simulink model "CATSS_Physical_ServiceCorePods"  (R2026a)
settings: Solver=VariableStepAuto
settings Model: DataDictionary=CATSS_PhysicalInterfaces.sldd  Creator=sdagen  LastModifiedBy=sdagen

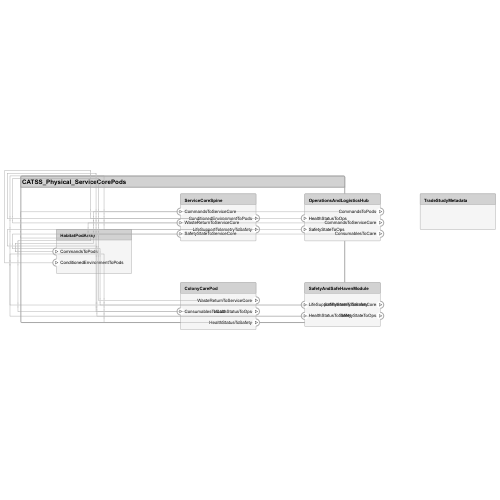
[thumbnail: Simulink's stored preview of the top-level diagram]
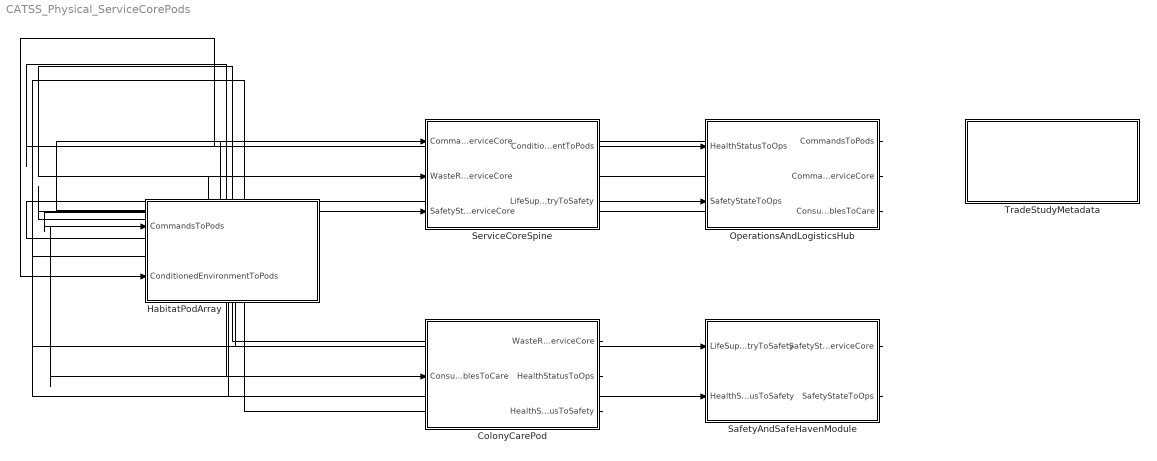
== system CATSS_Physical_ServiceCorePods ==
  ColonyCarePod : Subsystem
      settings: PortSchema="{\"entries\":[{\"content\":{\"headerSize\":26,\"margin\":15,\"minimumSpacing\":25,\"sides\":[{\"content\":{\"connectorIds\":[\"In1\"]},\"type\":\"ConnectorPlacement.EquallySpacedRectSide\",\"uuid\":\"fac29802-5ea5-4ebb-a4ed-86ec77815f5f\"},{\"content\":{\"connectorIds\":[\"Out1\",\"Out2\",\"Out3\"],\"side\":\"RIGHT\"},\"type\":\"ConnectorPlacement.EquallySpacedRectSide\",\"uuid\":\"7714f217-6bf1-4c7c-9160-bb80ade3ec0d\"},{\"content\":{\"side\":\"TOP\"},\"type\":\"ConnectorPlacement.EquallySpacedRectSide\",\"uuid\":\"21f04823-5172-4490-ad65-82ec45233f3c\"}]},\"type\":\"ConnectorPlacement.EquallySpacedConnector\",\"uuid\":\"7a688d36-5efc-41ce-92bb-92fe971cf983\"}],\"packageUris\":[\"http://schema.mathworks.com/mf0/Connector/R2020b\"],\"version\":\"1.0\"}"
  HabitatPodArray : Subsystem
      settings: PortSchema="{\"entries\":[{\"content\":{\"headerSize\":26,\"margin\":15,\"minimumSpacing\":25,\"sides\":[{\"content\":{\"connectorIds\":[\"In1\",\"In2\"]},\"type\":\"ConnectorPlacement.EquallySpacedRectSide\",\"uuid\":\"fac29802-5ea5-4ebb-a4ed-86ec77815f5f\"},{\"content\":{\"side\":\"RIGHT\"},\"type\":\"ConnectorPlacement.EquallySpacedRectSide\",\"uuid\":\"7714f217-6bf1-4c7c-9160-bb80ade3ec0d\"},{\"content\":{\"side\":\"TOP\"},\"type\":\"ConnectorPlacement.EquallySpacedRectSide\",\"uuid\":\"21f04823-5172-4490-ad65-82ec45233f3c\"}]},\"type\":\"ConnectorPlacement.EquallySpacedConnector\",\"uuid\":\"7a688d36-5efc-41ce-92bb-92fe971cf983\"}],\"packageUris\":[\"http://schema.mathworks.com/mf0/Connector/R2020b\"],\"version\":\"1.0\"}"
  OperationsAndLogisticsHub : Subsystem
      settings: PortSchema="{\"entries\":[{\"content\":{\"headerSize\":26,\"margin\":15,\"minimumSpacing\":25,\"sides\":[{\"content\":{\"connectorIds\":[\"In1\",\"In2\"]},\"type\":\"ConnectorPlacement.EquallySpacedRectSide\",\"uuid\":\"fac29802-5ea5-4ebb-a4ed-86ec77815f5f\"},{\"content\":{\"connectorIds\":[\"Out1\",\"Out2\",\"Out3\"],\"side\":\"RIGHT\"},\"type\":\"ConnectorPlacement.EquallySpacedRectSide\",\"uuid\":\"7714f217-6bf1-4c7c-9160-bb80ade3ec0d\"},{\"content\":{\"side\":\"TOP\"},\"type\":\"ConnectorPlacement.EquallySpacedRectSide\",\"uuid\":\"21f04823-5172-4490-ad65-82ec45233f3c\"}]},\"type\":\"ConnectorPlacement.EquallySpacedConnector\",\"uuid\":\"7a688d36-5efc-41ce-92bb-92fe971cf983\"}],\"packageUris\":[\"http://schema.mathworks.com/mf0/Connector/R2020b\"],\"version\":\"1.0\"}"
  SafetyAndSafeHavenModule : Subsystem
      settings: PortSchema="{\"entries\":[{\"content\":{\"headerSize\":26,\"margin\":15,\"minimumSpacing\":25,\"sides\":[{\"content\":{\"connectorIds\":[\"In1\",\"In2\"]},\"type\":\"ConnectorPlacement.EquallySpacedRectSide\",\"uuid\":\"fac29802-5ea5-4ebb-a4ed-86ec77815f5f\"},{\"content\":{\"connectorIds\":[\"Out1\",\"Out2\"],\"side\":\"RIGHT\"},\"type\":\"ConnectorPlacement.EquallySpacedRectSide\",\"uuid\":\"7714f217-6bf1-4c7c-9160-bb80ade3ec0d\"},{\"content\":{\"side\":\"TOP\"},\"type\":\"ConnectorPlacement.EquallySpacedRectSide\",\"uuid\":\"21f04823-5172-4490-ad65-82ec45233f3c\"}]},\"type\":\"ConnectorPlacement.EquallySpacedConnector\",\"uuid\":\"7a688d36-5efc-41ce-92bb-92fe971cf983\"}],\"packageUris\":[\"http://schema.mathworks.com/mf0/Connector/R2020b\"],\"version\":\"1.0\"}"
  ServiceCoreSpine : Subsystem
      settings: PortSchema="{\"entries\":[{\"content\":{\"headerSize\":26,\"margin\":15,\"minimumSpacing\":25,\"sides\":[{\"content\":{\"connectorIds\":[\"In1\",\"In2\",\"In3\"]},\"type\":\"ConnectorPlacement.EquallySpacedRectSide\",\"uuid\":\"fac29802-5ea5-4ebb-a4ed-86ec77815f5f\"},{\"content\":{\"connectorIds\":[\"Out1\",\"Out2\"],\"side\":\"RIGHT\"},\"type\":\"ConnectorPlacement.EquallySpacedRectSide\",\"uuid\":\"7714f217-6bf1-4c7c-9160-bb80ade3ec0d\"},{\"content\":{\"side\":\"TOP\"},\"type\":\"ConnectorPlacement.EquallySpacedRectSide\",\"uuid\":\"21f04823-5172-4490-ad65-82ec45233f3c\"}]},\"type\":\"ConnectorPlacement.EquallySpacedConnector\",\"uuid\":\"7a688d36-5efc-41ce-92bb-92fe971cf983\"}],\"packageUris\":[\"http://schema.mathworks.com/mf0/Connector/R2020b\"],\"version\":\"1.0\"}"
  TradeStudyMetadata : Subsystem
      settings: PortSchema="{\"entries\":[{\"content\":{\"headerSize\":26,\"margin\":15,\"minimumSpacing\":25,\"sides\":[{\"content\":{},\"type\":\"ConnectorPlacement.EquallySpacedRectSide\",\"uuid\":\"fac29802-5ea5-4ebb-a4ed-86ec77815f5f\"},{\"content\":{\"side\":\"RIGHT\"},\"type\":\"ConnectorPlacement.EquallySpacedRectSide\",\"uuid\":\"7714f217-6bf1-4c7c-9160-bb80ade3ec0d\"},{\"content\":{\"side\":\"TOP\"},\"type\":\"ConnectorPlacement.EquallySpacedRectSide\",\"uuid\":\"21f04823-5172-4490-ad65-82ec45233f3c\"}]},\"type\":\"ConnectorPlacement.EquallySpacedConnector\",\"uuid\":\"7a688d36-5efc-41ce-92bb-92fe971cf983\"}],\"packageUris\":[\"http://schema.mathworks.com/mf0/Connector/R2020b\"],\"version\":\"1.0\"}"
  wires:
  OperationsAndLogisticsHub/1(CommandsToPods) -> HabitatPodArray/1(CommandsToPods)
  OperationsAndLogisticsHub/2(CommandsToServiceCore) -> ServiceCoreSpine/1(CommandsToServiceCore)
  OperationsAndLogisticsHub/3(ConsumablesToCare) -> ColonyCarePod/1(ConsumablesToCare)
  ServiceCoreSpine/1(ConditionedEnvironmentToPods) -> HabitatPodArray/2(ConditionedEnvironmentToPods)
  ServiceCoreSpine/2(LifeSupportTelemetryToSafety) -> SafetyAndSafeHavenModule/1(LifeSupportTelemetryToSafety)
  ColonyCarePod/1(WasteReturnToServiceCore) -> ServiceCoreSpine/2(WasteReturnToServiceCore)
  ColonyCarePod/2(HealthStatusToOps) -> OperationsAndLogisticsHub/1(HealthStatusToOps)
  ColonyCarePod/3(HealthStatusToSafety) -> SafetyAndSafeHavenModule/2(HealthStatusToSafety)
  SafetyAndSafeHavenModule/1(SafetyStateToServiceCore) -> ServiceCoreSpine/3(SafetyStateToServiceCore)
  SafetyAndSafeHavenModule/2(SafetyStateToOps) -> OperationsAndLogisticsHub/2(SafetyStateToOps)

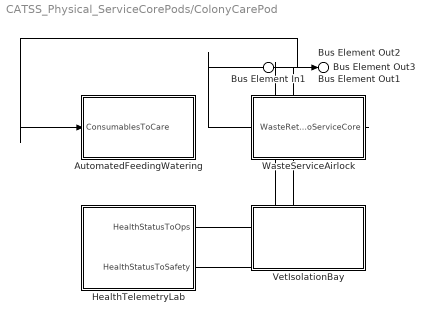
== system CATSS_Physical_ServiceCorePods/ColonyCarePod ==
  Bus Element In1 : Inport  PortName=ConsumablesToCare
  AutomatedFeedingWatering : Subsystem
      settings: PortSchema="{\"entries\":[{\"content\":{\"headerSize\":26,\"margin\":15,\"minimumSpacing\":25,\"sides\":[{\"content\":{\"connectorIds\":[\"In1\"]},\"type\":\"ConnectorPlacement.EquallySpacedRectSide\",\"uuid\":\"fac29802-5ea5-4ebb-a4ed-86ec77815f5f\"},{\"content\":{\"side\":\"RIGHT\"},\"type\":\"ConnectorPlacement.EquallySpacedRectSide\",\"uuid\":\"7714f217-6bf1-4c7c-9160-bb80ade3ec0d\"},{\"content\":{\"side\":\"TOP\"},\"type\":\"ConnectorPlacement.EquallySpacedRectSide\",\"uuid\":\"21f04823-5172-4490-ad65-82ec45233f3c\"}]},\"type\":\"ConnectorPlacement.EquallySpacedConnector\",\"uuid\":\"7a688d36-5efc-41ce-92bb-92fe971cf983\"}],\"packageUris\":[\"http://schema.mathworks.com/mf0/Connector/R2020b\"],\"version\":\"1.0\"}"
  HealthTelemetryLab : Subsystem
      settings: PortSchema="{\"entries\":[{\"content\":{\"headerSize\":26,\"margin\":15,\"minimumSpacing\":25,\"sides\":[{\"content\":{},\"type\":\"ConnectorPlacement.EquallySpacedRectSide\",\"uuid\":\"fac29802-5ea5-4ebb-a4ed-86ec77815f5f\"},{\"content\":{\"connectorIds\":[\"Out1\",\"Out2\"],\"side\":\"RIGHT\"},\"type\":\"ConnectorPlacement.EquallySpacedRectSide\",\"uuid\":\"7714f217-6bf1-4c7c-9160-bb80ade3ec0d\"},{\"content\":{\"side\":\"TOP\"},\"type\":\"ConnectorPlacement.EquallySpacedRectSide\",\"uuid\":\"21f04823-5172-4490-ad65-82ec45233f3c\"}]},\"type\":\"ConnectorPlacement.EquallySpacedConnector\",\"uuid\":\"7a688d36-5efc-41ce-92bb-92fe971cf983\"}],\"packageUris\":[\"http://schema.mathworks.com/mf0/Connector/R2020b\"],\"version\":\"1.0\"}"
  VetIsolationBay : Subsystem
      settings: PortSchema="{\"entries\":[{\"content\":{\"headerSize\":26,\"margin\":15,\"minimumSpacing\":25,\"sides\":[{\"content\":{},\"type\":\"ConnectorPlacement.EquallySpacedRectSide\",\"uuid\":\"fac29802-5ea5-4ebb-a4ed-86ec77815f5f\"},{\"content\":{\"side\":\"RIGHT\"},\"type\":\"ConnectorPlacement.EquallySpacedRectSide\",\"uuid\":\"7714f217-6bf1-4c7c-9160-bb80ade3ec0d\"},{\"content\":{\"side\":\"TOP\"},\"type\":\"ConnectorPlacement.EquallySpacedRectSide\",\"uuid\":\"21f04823-5172-4490-ad65-82ec45233f3c\"}]},\"type\":\"ConnectorPlacement.EquallySpacedConnector\",\"uuid\":\"7a688d36-5efc-41ce-92bb-92fe971cf983\"}],\"packageUris\":[\"http://schema.mathworks.com/mf0/Connector/R2020b\"],\"version\":\"1.0\"}"
  WasteServiceAirlock : Subsystem
      settings: PortSchema="{\"entries\":[{\"content\":{\"headerSize\":26,\"margin\":15,\"minimumSpacing\":25,\"sides\":[{\"content\":{},\"type\":\"ConnectorPlacement.EquallySpacedRectSide\",\"uuid\":\"fac29802-5ea5-4ebb-a4ed-86ec77815f5f\"},{\"content\":{\"connectorIds\":[\"Out1\"],\"side\":\"RIGHT\"},\"type\":\"ConnectorPlacement.EquallySpacedRectSide\",\"uuid\":\"7714f217-6bf1-4c7c-9160-bb80ade3ec0d\"},{\"content\":{\"side\":\"TOP\"},\"type\":\"ConnectorPlacement.EquallySpacedRectSide\",\"uuid\":\"21f04823-5172-4490-ad65-82ec45233f3c\"}]},\"type\":\"ConnectorPlacement.EquallySpacedConnector\",\"uuid\":\"7a688d36-5efc-41ce-92bb-92fe971cf983\"}],\"packageUris\":[\"http://schema.mathworks.com/mf0/Connector/R2020b\"],\"version\":\"1.0\"}"
  Bus Element Out1 : Outport  PortName=WasteReturnToServiceCore
  Bus Element Out2 : Outport  Port=2  PortName=HealthStatusToOps
  Bus Element Out3 : Outport  Port=3  PortName=HealthStatusToSafety
  wires:
  Bus Element In1/1 -> AutomatedFeedingWatering/1(ConsumablesToCare)
  HealthTelemetryLab/1(HealthStatusToOps) -> Bus Element Out2/1
  HealthTelemetryLab/2(HealthStatusToSafety) -> Bus Element Out3/1
  WasteServiceAirlock/1(WasteReturnToServiceCore) -> Bus Element Out1/1

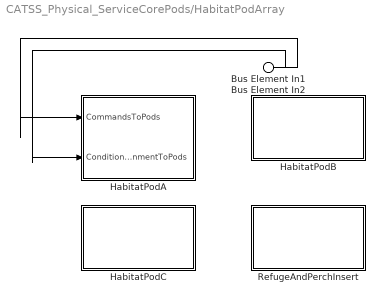
== system CATSS_Physical_ServiceCorePods/HabitatPodArray ==
  Bus Element In1 : Inport  PortName=CommandsToPods
  Bus Element In2 : Inport  Port=2  PortName=ConditionedEnvironmentToPods
  HabitatPodA : Subsystem
      settings: PortSchema="{\"entries\":[{\"content\":{\"headerSize\":26,\"margin\":15,\"minimumSpacing\":25,\"sides\":[{\"content\":{\"connectorIds\":[\"In1\",\"In2\"]},\"type\":\"ConnectorPlacement.EquallySpacedRectSide\",\"uuid\":\"fac29802-5ea5-4ebb-a4ed-86ec77815f5f\"},{\"content\":{\"side\":\"RIGHT\"},\"type\":\"ConnectorPlacement.EquallySpacedRectSide\",\"uuid\":\"7714f217-6bf1-4c7c-9160-bb80ade3ec0d\"},{\"content\":{\"side\":\"TOP\"},\"type\":\"ConnectorPlacement.EquallySpacedRectSide\",\"uuid\":\"21f04823-5172-4490-ad65-82ec45233f3c\"}]},\"type\":\"ConnectorPlacement.EquallySpacedConnector\",\"uuid\":\"7a688d36-5efc-41ce-92bb-92fe971cf983\"}],\"packageUris\":[\"http://schema.mathworks.com/mf0/Connector/R2020b\"],\"version\":\"1.0\"}"
  HabitatPodB : Subsystem
      settings: PortSchema="{\"entries\":[{\"content\":{\"headerSize\":26,\"margin\":15,\"minimumSpacing\":25,\"sides\":[{\"content\":{},\"type\":\"ConnectorPlacement.EquallySpacedRectSide\",\"uuid\":\"fac29802-5ea5-4ebb-a4ed-86ec77815f5f\"},{\"content\":{\"side\":\"RIGHT\"},\"type\":\"ConnectorPlacement.EquallySpacedRectSide\",\"uuid\":\"7714f217-6bf1-4c7c-9160-bb80ade3ec0d\"},{\"content\":{\"side\":\"TOP\"},\"type\":\"ConnectorPlacement.EquallySpacedRectSide\",\"uuid\":\"21f04823-5172-4490-ad65-82ec45233f3c\"}]},\"type\":\"ConnectorPlacement.EquallySpacedConnector\",\"uuid\":\"7a688d36-5efc-41ce-92bb-92fe971cf983\"}],\"packageUris\":[\"http://schema.mathworks.com/mf0/Connector/R2020b\"],\"version\":\"1.0\"}"
  HabitatPodC : Subsystem
      settings: PortSchema="{\"entries\":[{\"content\":{\"headerSize\":26,\"margin\":15,\"minimumSpacing\":25,\"sides\":[{\"content\":{},\"type\":\"ConnectorPlacement.EquallySpacedRectSide\",\"uuid\":\"fac29802-5ea5-4ebb-a4ed-86ec77815f5f\"},{\"content\":{\"side\":\"RIGHT\"},\"type\":\"ConnectorPlacement.EquallySpacedRectSide\",\"uuid\":\"7714f217-6bf1-4c7c-9160-bb80ade3ec0d\"},{\"content\":{\"side\":\"TOP\"},\"type\":\"ConnectorPlacement.EquallySpacedRectSide\",\"uuid\":\"21f04823-5172-4490-ad65-82ec45233f3c\"}]},\"type\":\"ConnectorPlacement.EquallySpacedConnector\",\"uuid\":\"7a688d36-5efc-41ce-92bb-92fe971cf983\"}],\"packageUris\":[\"http://schema.mathworks.com/mf0/Connector/R2020b\"],\"version\":\"1.0\"}"
  RefugeAndPerchInsert : Subsystem
      settings: PortSchema="{\"entries\":[{\"content\":{\"headerSize\":26,\"margin\":15,\"minimumSpacing\":25,\"sides\":[{\"content\":{},\"type\":\"ConnectorPlacement.EquallySpacedRectSide\",\"uuid\":\"fac29802-5ea5-4ebb-a4ed-86ec77815f5f\"},{\"content\":{\"side\":\"RIGHT\"},\"type\":\"ConnectorPlacement.EquallySpacedRectSide\",\"uuid\":\"7714f217-6bf1-4c7c-9160-bb80ade3ec0d\"},{\"content\":{\"side\":\"TOP\"},\"type\":\"ConnectorPlacement.EquallySpacedRectSide\",\"uuid\":\"21f04823-5172-4490-ad65-82ec45233f3c\"}]},\"type\":\"ConnectorPlacement.EquallySpacedConnector\",\"uuid\":\"7a688d36-5efc-41ce-92bb-92fe971cf983\"}],\"packageUris\":[\"http://schema.mathworks.com/mf0/Connector/R2020b\"],\"version\":\"1.0\"}"
  wires:
  Bus Element In1/1 -> HabitatPodA/1(CommandsToPods)
  Bus Element In2/1 -> HabitatPodA/2(ConditionedEnvironmentToPods)

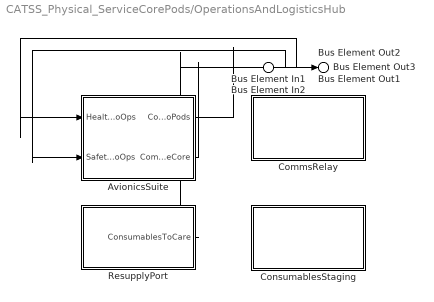
== system CATSS_Physical_ServiceCorePods/OperationsAndLogisticsHub ==
  Bus Element In1 : Inport  PortName=HealthStatusToOps
  Bus Element In2 : Inport  Port=2  PortName=SafetyStateToOps
  AvionicsSuite : Subsystem
      settings: PortSchema="{\"entries\":[{\"content\":{\"headerSize\":26,\"margin\":15,\"minimumSpacing\":25,\"sides\":[{\"content\":{\"connectorIds\":[\"In1\",\"In2\"]},\"type\":\"ConnectorPlacement.EquallySpacedRectSide\",\"uuid\":\"fac29802-5ea5-4ebb-a4ed-86ec77815f5f\"},{\"content\":{\"connectorIds\":[\"Out1\",\"Out2\"],\"side\":\"RIGHT\"},\"type\":\"ConnectorPlacement.EquallySpacedRectSide\",\"uuid\":\"7714f217-6bf1-4c7c-9160-bb80ade3ec0d\"},{\"content\":{\"side\":\"TOP\"},\"type\":\"ConnectorPlacement.EquallySpacedRectSide\",\"uuid\":\"21f04823-5172-4490-ad65-82ec45233f3c\"}]},\"type\":\"ConnectorPlacement.EquallySpacedConnector\",\"uuid\":\"7a688d36-5efc-41ce-92bb-92fe971cf983\"}],\"packageUris\":[\"http://schema.mathworks.com/mf0/Connector/R2020b\"],\"version\":\"1.0\"}"
  CommsRelay : Subsystem
      settings: PortSchema="{\"entries\":[{\"content\":{\"headerSize\":26,\"margin\":15,\"minimumSpacing\":25,\"sides\":[{\"content\":{},\"type\":\"ConnectorPlacement.EquallySpacedRectSide\",\"uuid\":\"fac29802-5ea5-4ebb-a4ed-86ec77815f5f\"},{\"content\":{\"side\":\"RIGHT\"},\"type\":\"ConnectorPlacement.EquallySpacedRectSide\",\"uuid\":\"7714f217-6bf1-4c7c-9160-bb80ade3ec0d\"},{\"content\":{\"side\":\"TOP\"},\"type\":\"ConnectorPlacement.EquallySpacedRectSide\",\"uuid\":\"21f04823-5172-4490-ad65-82ec45233f3c\"}]},\"type\":\"ConnectorPlacement.EquallySpacedConnector\",\"uuid\":\"7a688d36-5efc-41ce-92bb-92fe971cf983\"}],\"packageUris\":[\"http://schema.mathworks.com/mf0/Connector/R2020b\"],\"version\":\"1.0\"}"
  ConsumablesStaging : Subsystem
      settings: PortSchema="{\"entries\":[{\"content\":{\"headerSize\":26,\"margin\":15,\"minimumSpacing\":25,\"sides\":[{\"content\":{},\"type\":\"ConnectorPlacement.EquallySpacedRectSide\",\"uuid\":\"fac29802-5ea5-4ebb-a4ed-86ec77815f5f\"},{\"content\":{\"side\":\"RIGHT\"},\"type\":\"ConnectorPlacement.EquallySpacedRectSide\",\"uuid\":\"7714f217-6bf1-4c7c-9160-bb80ade3ec0d\"},{\"content\":{\"side\":\"TOP\"},\"type\":\"ConnectorPlacement.EquallySpacedRectSide\",\"uuid\":\"21f04823-5172-4490-ad65-82ec45233f3c\"}]},\"type\":\"ConnectorPlacement.EquallySpacedConnector\",\"uuid\":\"7a688d36-5efc-41ce-92bb-92fe971cf983\"}],\"packageUris\":[\"http://schema.mathworks.com/mf0/Connector/R2020b\"],\"version\":\"1.0\"}"
  ResupplyPort : Subsystem
      settings: PortSchema="{\"entries\":[{\"content\":{\"headerSize\":26,\"margin\":15,\"minimumSpacing\":25,\"sides\":[{\"content\":{},\"type\":\"ConnectorPlacement.EquallySpacedRectSide\",\"uuid\":\"fac29802-5ea5-4ebb-a4ed-86ec77815f5f\"},{\"content\":{\"connectorIds\":[\"Out1\"],\"side\":\"RIGHT\"},\"type\":\"ConnectorPlacement.EquallySpacedRectSide\",\"uuid\":\"7714f217-6bf1-4c7c-9160-bb80ade3ec0d\"},{\"content\":{\"side\":\"TOP\"},\"type\":\"ConnectorPlacement.EquallySpacedRectSide\",\"uuid\":\"21f04823-5172-4490-ad65-82ec45233f3c\"}]},\"type\":\"ConnectorPlacement.EquallySpacedConnector\",\"uuid\":\"7a688d36-5efc-41ce-92bb-92fe971cf983\"}],\"packageUris\":[\"http://schema.mathworks.com/mf0/Connector/R2020b\"],\"version\":\"1.0\"}"
  Bus Element Out1 : Outport  PortName=CommandsToPods
  Bus Element Out2 : Outport  Port=2  PortName=CommandsToServiceCore
  Bus Element Out3 : Outport  Port=3  PortName=ConsumablesToCare
  wires:
  AvionicsSuite/1(CommandsToPods) -> Bus Element Out1/1
  AvionicsSuite/2(CommandsToServiceCore) -> Bus Element Out2/1
  ResupplyPort/1(ConsumablesToCare) -> Bus Element Out3/1
  Bus Element In1/1 -> AvionicsSuite/1(HealthStatusToOps)
  Bus Element In2/1 -> AvionicsSuite/2(SafetyStateToOps)

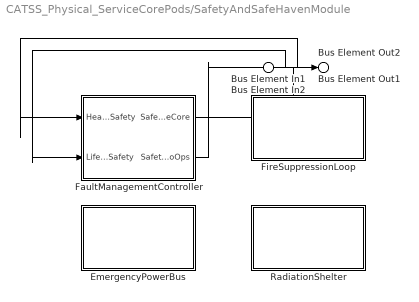
== system CATSS_Physical_ServiceCorePods/SafetyAndSafeHavenModule ==
  Bus Element In1 : Inport  PortName=LifeSupportTelemetryToSafety
  Bus Element In2 : Inport  Port=2  PortName=HealthStatusToSafety
  EmergencyPowerBus : Subsystem
      settings: PortSchema="{\"entries\":[{\"content\":{\"headerSize\":26,\"margin\":15,\"minimumSpacing\":25,\"sides\":[{\"content\":{},\"type\":\"ConnectorPlacement.EquallySpacedRectSide\",\"uuid\":\"fac29802-5ea5-4ebb-a4ed-86ec77815f5f\"},{\"content\":{\"side\":\"RIGHT\"},\"type\":\"ConnectorPlacement.EquallySpacedRectSide\",\"uuid\":\"7714f217-6bf1-4c7c-9160-bb80ade3ec0d\"},{\"content\":{\"side\":\"TOP\"},\"type\":\"ConnectorPlacement.EquallySpacedRectSide\",\"uuid\":\"21f04823-5172-4490-ad65-82ec45233f3c\"}]},\"type\":\"ConnectorPlacement.EquallySpacedConnector\",\"uuid\":\"7a688d36-5efc-41ce-92bb-92fe971cf983\"}],\"packageUris\":[\"http://schema.mathworks.com/mf0/Connector/R2020b\"],\"version\":\"1.0\"}"
  FaultManagementController : Subsystem
      settings: PortSchema="{\"entries\":[{\"content\":{\"headerSize\":26,\"margin\":15,\"minimumSpacing\":25,\"sides\":[{\"content\":{\"connectorIds\":[\"In1\",\"In2\"]},\"type\":\"ConnectorPlacement.EquallySpacedRectSide\",\"uuid\":\"fac29802-5ea5-4ebb-a4ed-86ec77815f5f\"},{\"content\":{\"connectorIds\":[\"Out1\",\"Out2\"],\"side\":\"RIGHT\"},\"type\":\"ConnectorPlacement.EquallySpacedRectSide\",\"uuid\":\"7714f217-6bf1-4c7c-9160-bb80ade3ec0d\"},{\"content\":{\"side\":\"TOP\"},\"type\":\"ConnectorPlacement.EquallySpacedRectSide\",\"uuid\":\"21f04823-5172-4490-ad65-82ec45233f3c\"}]},\"type\":\"ConnectorPlacement.EquallySpacedConnector\",\"uuid\":\"7a688d36-5efc-41ce-92bb-92fe971cf983\"}],\"packageUris\":[\"http://schema.mathworks.com/mf0/Connector/R2020b\"],\"version\":\"1.0\"}"
  FireSuppressionLoop : Subsystem
      settings: PortSchema="{\"entries\":[{\"content\":{\"headerSize\":26,\"margin\":15,\"minimumSpacing\":25,\"sides\":[{\"content\":{},\"type\":\"ConnectorPlacement.EquallySpacedRectSide\",\"uuid\":\"fac29802-5ea5-4ebb-a4ed-86ec77815f5f\"},{\"content\":{\"side\":\"RIGHT\"},\"type\":\"ConnectorPlacement.EquallySpacedRectSide\",\"uuid\":\"7714f217-6bf1-4c7c-9160-bb80ade3ec0d\"},{\"content\":{\"side\":\"TOP\"},\"type\":\"ConnectorPlacement.EquallySpacedRectSide\",\"uuid\":\"21f04823-5172-4490-ad65-82ec45233f3c\"}]},\"type\":\"ConnectorPlacement.EquallySpacedConnector\",\"uuid\":\"7a688d36-5efc-41ce-92bb-92fe971cf983\"}],\"packageUris\":[\"http://schema.mathworks.com/mf0/Connector/R2020b\"],\"version\":\"1.0\"}"
  RadiationShelter : Subsystem
      settings: PortSchema="{\"entries\":[{\"content\":{\"headerSize\":26,\"margin\":15,\"minimumSpacing\":25,\"sides\":[{\"content\":{},\"type\":\"ConnectorPlacement.EquallySpacedRectSide\",\"uuid\":\"fac29802-5ea5-4ebb-a4ed-86ec77815f5f\"},{\"content\":{\"side\":\"RIGHT\"},\"type\":\"ConnectorPlacement.EquallySpacedRectSide\",\"uuid\":\"7714f217-6bf1-4c7c-9160-bb80ade3ec0d\"},{\"content\":{\"side\":\"TOP\"},\"type\":\"ConnectorPlacement.EquallySpacedRectSide\",\"uuid\":\"21f04823-5172-4490-ad65-82ec45233f3c\"}]},\"type\":\"ConnectorPlacement.EquallySpacedConnector\",\"uuid\":\"7a688d36-5efc-41ce-92bb-92fe971cf983\"}],\"packageUris\":[\"http://schema.mathworks.com/mf0/Connector/R2020b\"],\"version\":\"1.0\"}"
  Bus Element Out1 : Outport  PortName=SafetyStateToServiceCore
  Bus Element Out2 : Outport  Port=2  PortName=SafetyStateToOps
  wires:
  Bus Element In2/1 -> FaultManagementController/1(HealthStatusToSafety)
  Bus Element In1/1 -> FaultManagementController/2(LifeSupportTelemetryToSafety)
  FaultManagementController/1(SafetyStateToServiceCore) -> Bus Element Out1/1
  FaultManagementController/2(SafetyStateToOps) -> Bus Element Out2/1

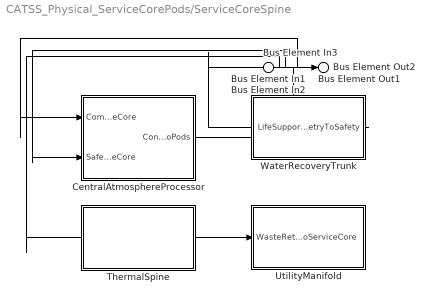
== system CATSS_Physical_ServiceCorePods/ServiceCoreSpine ==
  Bus Element In1 : Inport  PortName=CommandsToServiceCore
  Bus Element In2 : Inport  Port=2  PortName=WasteReturnToServiceCore
  Bus Element In3 : Inport  Port=3  PortName=SafetyStateToServiceCore
  CentralAtmosphereProcessor : Subsystem
      settings: PortSchema="{\"entries\":[{\"content\":{\"headerSize\":26,\"margin\":15,\"minimumSpacing\":25,\"sides\":[{\"content\":{\"connectorIds\":[\"In1\",\"In2\"]},\"type\":\"ConnectorPlacement.EquallySpacedRectSide\",\"uuid\":\"fac29802-5ea5-4ebb-a4ed-86ec77815f5f\"},{\"content\":{\"connectorIds\":[\"Out1\"],\"side\":\"RIGHT\"},\"type\":\"ConnectorPlacement.EquallySpacedRectSide\",\"uuid\":\"7714f217-6bf1-4c7c-9160-bb80ade3ec0d\"},{\"content\":{\"side\":\"TOP\"},\"type\":\"ConnectorPlacement.EquallySpacedRectSide\",\"uuid\":\"21f04823-5172-4490-ad65-82ec45233f3c\"}]},\"type\":\"ConnectorPlacement.EquallySpacedConnector\",\"uuid\":\"7a688d36-5efc-41ce-92bb-92fe971cf983\"}],\"packageUris\":[\"http://schema.mathworks.com/mf0/Connector/R2020b\"],\"version\":\"1.0\"}"
  ThermalSpine : Subsystem
      settings: PortSchema="{\"entries\":[{\"content\":{\"headerSize\":26,\"margin\":15,\"minimumSpacing\":25,\"sides\":[{\"content\":{},\"type\":\"ConnectorPlacement.EquallySpacedRectSide\",\"uuid\":\"fac29802-5ea5-4ebb-a4ed-86ec77815f5f\"},{\"content\":{\"side\":\"RIGHT\"},\"type\":\"ConnectorPlacement.EquallySpacedRectSide\",\"uuid\":\"7714f217-6bf1-4c7c-9160-bb80ade3ec0d\"},{\"content\":{\"side\":\"TOP\"},\"type\":\"ConnectorPlacement.EquallySpacedRectSide\",\"uuid\":\"21f04823-5172-4490-ad65-82ec45233f3c\"}]},\"type\":\"ConnectorPlacement.EquallySpacedConnector\",\"uuid\":\"7a688d36-5efc-41ce-92bb-92fe971cf983\"}],\"packageUris\":[\"http://schema.mathworks.com/mf0/Connector/R2020b\"],\"version\":\"1.0\"}"
  UtilityManifold : Subsystem
      settings: PortSchema="{\"entries\":[{\"content\":{\"headerSize\":26,\"margin\":15,\"minimumSpacing\":25,\"sides\":[{\"content\":{\"connectorIds\":[\"In1\"]},\"type\":\"ConnectorPlacement.EquallySpacedRectSide\",\"uuid\":\"fac29802-5ea5-4ebb-a4ed-86ec77815f5f\"},{\"content\":{\"side\":\"RIGHT\"},\"type\":\"ConnectorPlacement.EquallySpacedRectSide\",\"uuid\":\"7714f217-6bf1-4c7c-9160-bb80ade3ec0d\"},{\"content\":{\"side\":\"TOP\"},\"type\":\"ConnectorPlacement.EquallySpacedRectSide\",\"uuid\":\"21f04823-5172-4490-ad65-82ec45233f3c\"}]},\"type\":\"ConnectorPlacement.EquallySpacedConnector\",\"uuid\":\"7a688d36-5efc-41ce-92bb-92fe971cf983\"}],\"packageUris\":[\"http://schema.mathworks.com/mf0/Connector/R2020b\"],\"version\":\"1.0\"}"
  WaterRecoveryTrunk : Subsystem
      settings: PortSchema="{\"entries\":[{\"content\":{\"headerSize\":26,\"margin\":15,\"minimumSpacing\":25,\"sides\":[{\"content\":{},\"type\":\"ConnectorPlacement.EquallySpacedRectSide\",\"uuid\":\"fac29802-5ea5-4ebb-a4ed-86ec77815f5f\"},{\"content\":{\"connectorIds\":[\"Out1\"],\"side\":\"RIGHT\"},\"type\":\"ConnectorPlacement.EquallySpacedRectSide\",\"uuid\":\"7714f217-6bf1-4c7c-9160-bb80ade3ec0d\"},{\"content\":{\"side\":\"TOP\"},\"type\":\"ConnectorPlacement.EquallySpacedRectSide\",\"uuid\":\"21f04823-5172-4490-ad65-82ec45233f3c\"}]},\"type\":\"ConnectorPlacement.EquallySpacedConnector\",\"uuid\":\"7a688d36-5efc-41ce-92bb-92fe971cf983\"}],\"packageUris\":[\"http://schema.mathworks.com/mf0/Connector/R2020b\"],\"version\":\"1.0\"}"
  Bus Element Out1 : Outport  PortName=ConditionedEnvironmentToPods
  Bus Element Out2 : Outport  Port=2  PortName=LifeSupportTelemetryToSafety
  wires:
  Bus Element In1/1 -> CentralAtmosphereProcessor/1(CommandsToServiceCore)
  Bus Element In3/1 -> CentralAtmosphereProcessor/2(SafetyStateToServiceCore)
  Bus Element In2/1 -> UtilityManifold/1(WasteReturnToServiceCore)
  CentralAtmosphereProcessor/1(ConditionedEnvironmentToPods) -> Bus Element Out1/1
  WaterRecoveryTrunk/1(LifeSupportTelemetryToSafety) -> Bus Element Out2/1

== system CATSS_Physical_ServiceCorePods/TradeStudyMetadata ==

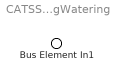
== system CATSS_Physical_ServiceCorePods/ColonyCarePod/AutomatedFeedingWatering ==
  Bus Element In1 : Inport  PortName=ConsumablesToCare

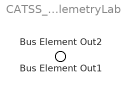
== system CATSS_Physical_ServiceCorePods/ColonyCarePod/HealthTelemetryLab ==
  Bus Element Out1 : Outport  PortName=HealthStatusToOps
  Bus Element Out2 : Outport  Port=2  PortName=HealthStatusToSafety

== system CATSS_Physical_ServiceCorePods/ColonyCarePod/VetIsolationBay ==

== system CATSS_Physical_ServiceCorePods/ColonyCarePod/WasteServiceAirlock ==
  Bus Element Out1 : Outport  PortName=WasteReturnToServiceCore

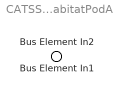
== system CATSS_Physical_ServiceCorePods/HabitatPodArray/HabitatPodA ==
  Bus Element In1 : Inport  PortName=CommandsToPods
  Bus Element In2 : Inport  Port=2  PortName=ConditionedEnvironmentToPods

== system CATSS_Physical_ServiceCorePods/HabitatPodArray/HabitatPodB ==

== system CATSS_Physical_ServiceCorePods/HabitatPodArray/HabitatPodC ==

== system CATSS_Physical_ServiceCorePods/HabitatPodArray/RefugeAndPerchInsert ==

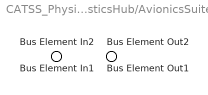
== system CATSS_Physical_ServiceCorePods/OperationsAndLogisticsHub/AvionicsSuite ==
  Bus Element In1 : Inport  PortName=HealthStatusToOps
  Bus Element In2 : Inport  Port=2  PortName=SafetyStateToOps
  Bus Element Out1 : Outport  PortName=CommandsToPods
  Bus Element Out2 : Outport  Port=2  PortName=CommandsToServiceCore

== system CATSS_Physical_ServiceCorePods/OperationsAndLogisticsHub/CommsRelay ==

== system CATSS_Physical_ServiceCorePods/OperationsAndLogisticsHub/ConsumablesStaging ==

== system CATSS_Physical_ServiceCorePods/OperationsAndLogisticsHub/ResupplyPort ==
  Bus Element Out1 : Outport  PortName=ConsumablesToCare

== system CATSS_Physical_ServiceCorePods/SafetyAndSafeHavenModule/EmergencyPowerBus ==

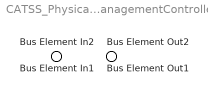
== system CATSS_Physical_ServiceCorePods/SafetyAndSafeHavenModule/FaultManagementController ==
  Bus Element In1 : Inport  PortName=HealthStatusToSafety
  Bus Element In2 : Inport  Port=2  PortName=LifeSupportTelemetryToSafety
  Bus Element Out1 : Outport  PortName=SafetyStateToServiceCore
  Bus Element Out2 : Outport  Port=2  PortName=SafetyStateToOps

== system CATSS_Physical_ServiceCorePods/SafetyAndSafeHavenModule/FireSuppressionLoop ==

== system CATSS_Physical_ServiceCorePods/SafetyAndSafeHavenModule/RadiationShelter ==

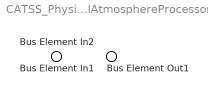
== system CATSS_Physical_ServiceCorePods/ServiceCoreSpine/CentralAtmosphereProcessor ==
  Bus Element In1 : Inport  PortName=CommandsToServiceCore
  Bus Element In2 : Inport  Port=2  PortName=SafetyStateToServiceCore
  Bus Element Out1 : Outport  PortName=ConditionedEnvironmentToPods

== system CATSS_Physical_ServiceCorePods/ServiceCoreSpine/ThermalSpine ==

== system CATSS_Physical_ServiceCorePods/ServiceCoreSpine/UtilityManifold ==
  Bus Element In1 : Inport  PortName=WasteReturnToServiceCore

== system CATSS_Physical_ServiceCorePods/ServiceCoreSpine/WaterRecoveryTrunk ==
  Bus Element Out1 : Outport  PortName=LifeSupportTelemetryToSafety
